simulink model "actuador_modelo_global_NL"  (R2023b)
settings: Solver=VariableStepAuto  StartTime=0.0  StopTime=10.0  RelTol=1e-3
values from neighbouring files (symbols this model uses):
  alpha_Cu = 3.9e-3    (= 0.0039)    [controlador_foc_simulink.m]    (also in parametros_planta.m; params_subsistema_termico.m; sistema_completo_en_codigo.m)
  beq_nom = bm + bl_nom/r^2    (= 2.19444444444e-05)    [parametros_planta.m]    (also in params_subsistema_mecanico.m; sistema_completo_en_codigo.m)
  Cts = 0.818    [parametros_planta.m]    (also in params_subsistema_termico.m)
  Jeq_nom = Jm + Jl_nom/r^2    (= 1.97847222222e-05)    [params_subsistema_mecanico.m]    (also in sistema_completo_en_codigo.m)
  kg_eq_nom = g*kl_nom/r    (= 0.0204305208333)    [params_subsistema_mecanico.m]    (also in sistema_completo_en_codigo.m)
  L_d = 6.6e-3    (= 0.0066)    [controlador_foc_simulink.m]    (also in params_subsistema_electromagnetico.m; sistema_completo_en_codigo.m)
  L_l = 0.8e-3    (= 0.0008)    [controlador_foc_simulink.m]    (also in params_subsistema_electromagnetico.m; sistema_completo_en_codigo.m)
  L_q = 5.8e-3    (= 0.0058)    [controlador_foc_simulink.m]    (also in params_subsistema_electromagnetico.m; sistema_completo_en_codigo.m)
  lambda_m = 0.016    [controlador_foc_simulink.m]    (also in parametros_planta.m; params_subsistema_electromagnetico.m; sistema_completo_en_codigo.m)
  Pp = 3    [controlador_foc_simulink.m]    (also in parametros_planta.m; params_subsistema_electromagnetico.m; sistema_completo_en_codigo.m)
  r = 120.0    (= 120)    [controlador_foc_simulink.m]    (also in parametros_planta.m; params_subsistema_mecanico.m; sistema_completo_en_codigo.m)
  Rs_REF = 1.02    [controlador_foc_simulink.m]    (also in parametros_planta.m; params_subsistema_termico.m; sistema_completo_en_codigo.m)
  Rts_amb = 146.7    [parametros_planta.m]    (also in params_subsistema_termico.m)
  Tamb = Tamb_max    (= 40)    [parametros_planta.m]    (also in params_subsistema_termico.m; sistema_completo_en_codigo.m)
  Ts_REF = 20.0    (= 20)    [controlador_foc_simulink.m]    (also in parametros_planta.m; params_subsistema_termico.m; sistema_completo_en_codigo.m)
settings Model: Creator=Pc  LastModifiedBy=Gabriel

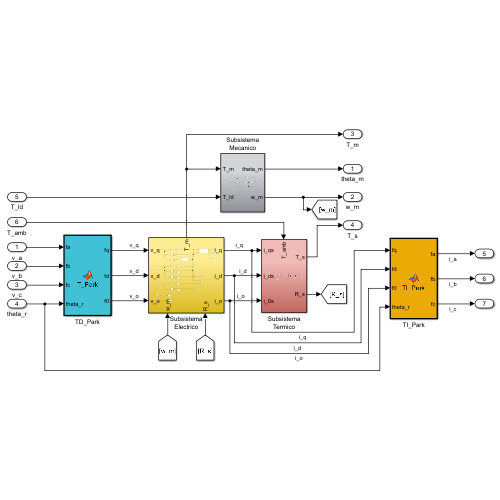
[thumbnail: Simulink's stored preview of the top-level diagram]
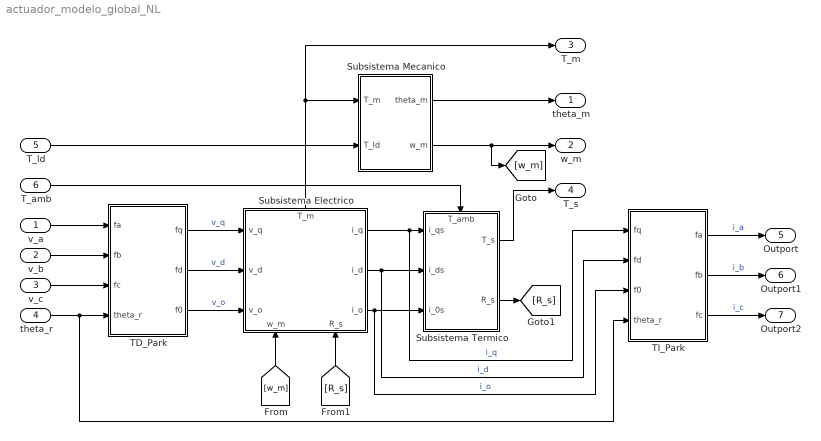
== system actuador_modelo_global_NL ==
  v_a : Inport
  v_b : Inport  Port=2
  v_c : Inport  Port=3
  theta_r : Inport  Port=4
  T_ld : Inport  Port=5
  T_amb : Inport  Port=6
  Subsistema Electrico : Subsystem
      settings: PortSchema="{\"entries\":[{\"content\":{\"sides\":[{\"content\":{\"connectorIds\":[\"In1\",\"In2\",\"In3\"]},\"type\":\"ConnectorPlacement.EquallySpacedRectSide\",\"uuid\":\"c7eb63ae-4015-4be9-a2f8-5ddbad38e871\"},{\"content\":{\"connectorIds\":[\"Out1\",\"Out2\",\"Out3\"],\"side\":\"RIGHT\"},\"type\":\"ConnectorPlacement.EquallySpacedRectSide\",\"uuid\":\"ed205027-9864-417a-9d2b-6eeb723ffec2\"},{\"content\":{\"connectorIds\":[\"Out4\"],\"side\":\"TOP\"},\"type\":\"ConnectorPlacement.EquallySpacedRectSide\",\"uuid\":\"5c5dee03-5728-4212-8fc2-a453d3484329\"},{\"content\":{\"connectorIds\":[\"In4\",\"In5\"],\"side\":\"BOTTOM\"},\"type\":\"ConnectorPlacement.EquallySpacedRectSide\",\"uuid\":\"494df340-b6d5-4f09-932e-9dbff39af1cf\"}]},\"type\":\"ConnectorPlacement.EquallySpacedConnector\",\"uuid\":\"0eeaea4c-3d80-4ebb-8c27-59b1b18764e9\"}],\"packageUris\":[\"http://schema.mathworks.com/mf0/Connector/R2020b\"],\"version\":\"1.0\"}"
  Subsistema Mecanico : Subsystem
  Subsistema Termico : Subsystem
      settings: PortSchema="{\"entries\":[{\"content\":{\"sides\":[{\"content\":{\"connectorIds\":[\"In1\",\"In2\",\"In3\"]},\"type\":\"ConnectorPlacement.EquallySpacedRectSide\",\"uuid\":\"5b1848a7-84bd-4673-a3fa-3976b4d0d5b9\"},{\"content\":{\"connectorIds\":[\"Out1\",\"Out2\"],\"side\":\"RIGHT\"},\"type\":\"ConnectorPlacement.EquallySpacedRectSide\",\"uuid\":\"feff3f8a-cd7c-43b1-91c3-7ab01b0b33a6\"},{\"content\":{\"connectorIds\":[\"In4\"],\"side\":\"TOP\"},\"type\":\"ConnectorPlacement.EquallySpacedRectSide\",\"uuid\":\"8de0b1b6-142f-442a-a92f-2baa615c6322\"}]},\"type\":\"ConnectorPlacement.EquallySpacedConnector\",\"uuid\":\"046fcb24-e0d9-4784-a784-7e36f9acbfbc\"}],\"packageUris\":[\"http://schema.mathworks.com/mf0/Connector/R2020b\"],\"version\":\"1.0\"}"
  TD_Park : MATLAB Function  TreatAsAtomicUnit=on
  TI_Park : MATLAB Function  TreatAsAtomicUnit=on
  theta_m : Outport
  w_m : Outport  Port=2
  T_m : Outport  Port=3
  T_s : Outport  Port=4
  Outport : Outport  Port=5
  Outport1 : Outport  Port=6
  Outport2 : Outport  Port=7
  wires:
  Subsistema Electrico/1(i_q) -> TI_Park/1(fq), Subsistema Termico/1(i_qs)  "i_q"
  Subsistema Electrico/2(i_d) -> Subsistema Termico/2(i_ds), TI_Park/2(fd)  "i_d"
  Subsistema Electrico/3(i_o) -> Subsistema Termico/3(i_0s), TI_Park/3(f0)  "i_o"
  TD_Park/1(fq) -> Subsistema Electrico/1(v_q)  "v_q"
  TD_Park/2(fd) -> Subsistema Electrico/2(v_d)  "v_d"
  TD_Park/3(f0) -> Subsistema Electrico/3(v_o)  "v_o"
  T_amb/1 -> Subsistema Termico/4(T_amb)
  Subsistema Mecanico/2(w_m) -> [w_m], w_m/1
  Subsistema Mecanico/1(theta_m) -> theta_m/1
  v_a/1 -> TD_Park/1(fa)
  v_b/1 -> TD_Park/2(fb)
  v_c/1 -> TD_Park/3(fc)
  Subsistema Termico/1(T_s) -> T_s/1
  theta_r/1 -> TI_Park/4(theta_r), TD_Park/4(theta_r)
  Subsistema Electrico/4(T_m) -> T_m/1, Subsistema Mecanico/1(T_m)
  T_ld/1 -> Subsistema Mecanico/2(T_ld)
  [w_m] -> Subsistema Electrico/4(w_m)
  Subsistema Termico/2(R_s) -> [R_s]
  [R_s] -> Subsistema Electrico/5(R_s)
  TI_Park/1(fa) -> Outport/1  "i_a"
  TI_Park/2(fb) -> Outport1/1  "i_b"
  TI_Park/3(fc) -> Outport2/1  "i_c"

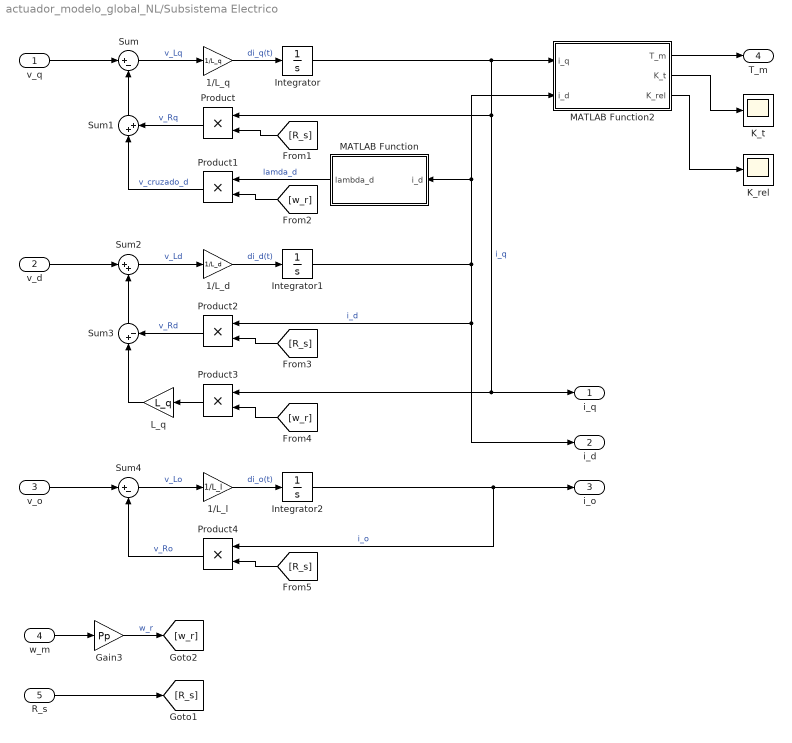
== system actuador_modelo_global_NL/Subsistema Electrico ==
  v_q : Inport
  v_d : Inport  Port=2
  v_o : Inport  Port=3
  w_m : Inport  Port=4
  R_s : Inport  Port=5
  1/L_d : Gain  Gain=1/L_d
  1/L_l : Gain  Gain=1/L_l
  1/L_q : Gain  Gain=1/L_q
  Gain3 : Gain  Gain=Pp
  Integrator : Integrator
  Integrator1 : Integrator
  Integrator2 : Integrator
  K_rel : Scope
  K_t : Scope
  L_q : Gain  Gain=L_q
  MATLAB Function : MATLAB Function  TreatAsAtomicUnit=on
  MATLAB Function2 : MATLAB Function  TreatAsAtomicUnit=on
  Product{,1..4} (5 alike) : Product
  Sum : Sum  Inputs=|+-
  Sum1 : Sum  Inputs=|++
  Sum2 : Sum  Inputs=|++
  Sum3 : Sum  Inputs=|+-
  Sum4 : Sum  Inputs=|+-
  i_q : Outport
  i_d : Outport  Port=2
  i_o : Outport  Port=3
  T_m : Outport  Port=4
  wires:
  Integrator/1 -> MATLAB Function2/1(i_q), Product/1, i_q/1, Product3/1  "i_q"
  Sum3/1 -> Sum2/2
  Product1/1 -> Sum1/1  "v_cruzado_d"
  Integrator1/1 -> MATLAB Function2/2(i_d), MATLAB Function/1(i_d), i_d/1, Product2/1  "i_d"
  Sum1/1 -> Sum/2
  1/L_d/1 -> Integrator1/1  "di_d(t)"
  MATLAB Function/1(lambda_d) -> Product1/1  "lamda_d"
  Sum4/1 -> 1/L_l/1  "v_Lo"
  [w_r] -> Product3/2
  Sum/1 -> 1/L_q/1  "v_Lq"
  1/L_l/1 -> Integrator2/1  "di_o(t)"
  Integrator2/1 -> i_o/1, Product4/1  "i_o"
  Product2/1 -> Sum3/2  "v_Rd"
  Product/1 -> Sum1/2  "v_Rq"
  [R_s] -> Product4/2
  Product3/1 -> L_q/1
  1/L_q/1 -> Integrator/1  "di_q(t)"
  Sum2/1 -> 1/L_d/1  "v_Ld"
  v_q/1 -> Sum/1
  [R_s] -> Product/2
  Product4/1 -> Sum4/2  "v_Ro"
  [w_r] -> Product1/2
  [R_s] -> Product2/2
  L_q/1 -> Sum3/1
  v_d/1 -> Sum2/1
  v_o/1 -> Sum4/1
  MATLAB Function2/1(T_m) -> T_m/1
  MATLAB Function2/3(K_rel) -> K_rel/1
  MATLAB Function2/2(K_t) -> K_t/1
  w_m/1 -> Gain3/1
  R_s/1 -> [R_s]
  Gain3/1 -> [w_r]  "w_r"

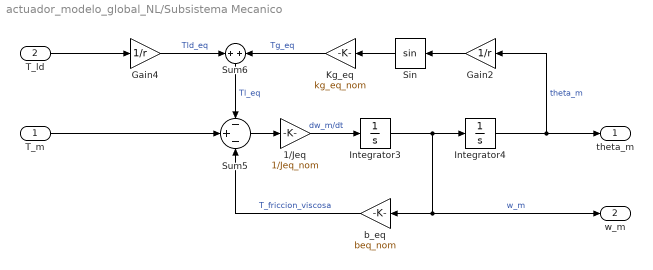
== system actuador_modelo_global_NL/Subsistema Mecanico ==
  T_m : Inport
  T_ld : Inport  Port=2
  1/Jeq : Gain  Gain=1/Jeq_nom
  Gain2 : Gain  Gain=1/r
  Gain4 : Gain  Gain=1/r
  Integrator3 : Integrator
  Integrator4 : Integrator
  Kg_eq : Gain  Gain=kg_eq_nom
  Sin : Trigonometry
  Sum5 : Sum  Inputs=-+-
  Sum6 : Sum  Inputs=+|+
  b_eq : Gain  Gain=beq_nom
  theta_m : Outport
  w_m : Outport  Port=2
  wires:
  Sin/1 -> Kg_eq/1
  Gain4/1 -> Sum6/1  "Tld_eq"
  Integrator4/1 -> theta_m/1, Gain2/1  "theta_m"
  Kg_eq/1 -> Sum6/2  "Tg_eq"
  Sum5/1 -> 1/Jeq/1
  b_eq/1 -> Sum5/3  "T_friccion_viscosa"
  T_m/1 -> Sum5/2
  Gain2/1 -> Sin/1
  Sum6/1 -> Sum5/1  "Tl_eq"
  Integrator3/1 -> w_m/1, b_eq/1, Integrator4/1  "w_m"
  T_ld/1 -> Gain4/1
  1/Jeq/1 -> Integrator3/1  "dw_m/dt"

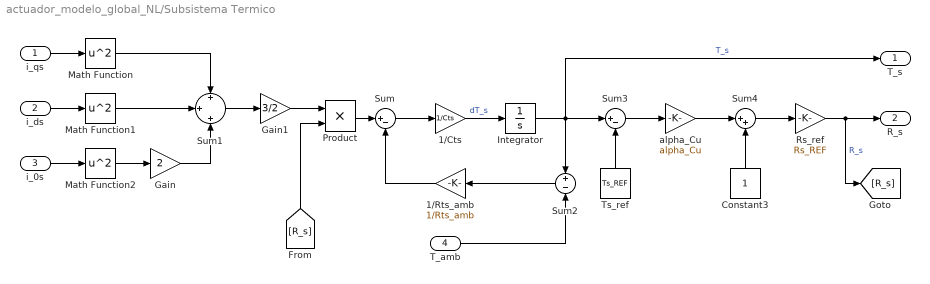
== system actuador_modelo_global_NL/Subsistema Termico ==
  i_qs : Inport
  i_ds : Inport  Port=2
  i_0s : Inport  Port=3
  T_amb : Inport  Port=4
  1/Cts : Gain  Gain=1/Cts
  1/Rts_amb : Gain  Gain=1/Rts_amb
  Constant3 : Constant
  Gain : Gain  Gain=2
  Gain1 : Gain  Gain=3/2
  Integrator : Integrator  InitialCondition=Tamb
  Math Function : Math  Operator=square
  Math Function1 : Math  Operator=square
  Math Function2 : Math  Operator=square
  Product : Product
  Rs_ref : Gain  Gain=Rs_REF
  Sum : Sum  Inputs=|+-
  Sum1 : Sum  Inputs=+|+|+
  Sum2 : Sum  Inputs=+-
  Sum3 : Sum  Inputs=|+-
  Sum4 : Sum  Inputs=|++
  Ts_ref : Constant  Value=Ts_REF
  alpha_Cu : Gain  Gain=alpha_Cu
  T_s : Outport
  R_s : Outport  Port=2
  wires:
  1/Cts/1 -> Integrator/1  "dT_s"
  Sum3/1 -> alpha_Cu/1
  Rs_ref/1 -> R_s/1, [R_s]  "R_s"
  Sum4/1 -> Rs_ref/1
  [R_s] -> Product/2
  i_ds/1 -> Math Function1/1
  Constant3/1 -> Sum4/2
  Integrator/1 -> T_s/1, Sum2/1, Sum3/1  "T_s"
  Math Function1/1 -> Sum1/2
  alpha_Cu/1 -> Sum4/1
  Sum2/1 -> 1/Rts_amb/1
  Product/1 -> Sum/1
  i_qs/1 -> Math Function/1
  Sum/1 -> 1/Cts/1
  T_amb/1 -> Sum2/2
  Math Function/1 -> Sum1/1
  i_0s/1 -> Math Function2/1
  1/Rts_amb/1 -> Sum/2
  Ts_ref/1 -> Sum3/2
  Math Function2/1 -> Gain/1
  Gain/1 -> Sum1/3
  Sum1/1 -> Gain1/1
  Gain1/1 -> Product/1

== matlab function actuador_modelo_global_NL/TD_Park ==
  data: fa input; fq output; fb input; fc input; theta_r input; fd output; f0 output
function [fq, fd, f0] = T_Park(fa, fb, fc, theta_r)
%#codegen
% Transformada directa de Park: abc -> qd0
% Convención usada:
% fq: eje q
% fd: eje d
% f0: componente homopolar

c1 = cos(theta_r);
c2 = cos(theta_r - 2*pi/3);
c3 = cos(theta_r + 2*pi/3);

s1 = sin(theta_r);
s2 = sin(theta_r - 2*pi/3);
s3 = sin(theta_r + 2*pi/3);

fq = (2/3)*(c1*fa + c2*fb + c3*fc);
fd = (2/3)*(s1*fa + s2*fb + s3*fc);
f0 = (1/3)*(fa + fb + fc);
end

== matlab function actuador_modelo_global_NL/Subsistema Electrico/MATLAB Function ==
  data: i_d input; lambda_d output; lambda_m parameter; L_d parameter
function lambda_d = calcular_flujo_d(i_d, lambda_m, L_d)
    % CALCULAR_FLUJO_D Calcula el flujo magnético total concatenado en el eje directo (d).
    %
    % Entradas:
    %   i_d      : Corriente instantánea en el eje d (Señal dinámica de entrada).
    %   lambda_m : Flujo de los imanes permanentes (Parámetro estático).
    %   L_d      : Inductancia del estator en el eje d (Parámetro estático).
    %
    % Salida:
    %   lambda_d : Flujo magnético total en el eje d.

    % Cálculo: Flujo de imanes + Flujo de reacción del inducido
    lambda_d = lambda_m + L_d * i_d;
end

== matlab function actuador_modelo_global_NL/Subsistema Electrico/MATLAB Function2 ==
  data: i_q input; i_d input; T_m output; Pp parameter; lambda_m parameter; L_d parameter; L_q parameter; K_t output; K_rel output
function [T_m, K_t, K_rel] = calcular_torque(i_q, i_d, Pp, lambda_m, L_d, L_q)
    % CALCULAR_TORQUE Calcula el torque electromagnético total de la máquina PMSM
    % y sus constantes equivalentes.
    % 
    % Entradas dinámicas (Inports):
    %   i_q      : Corriente en el eje en cuadratura [A].
    %   i_d      : Corriente en el eje directo [A].
    %
    % Parámetros estáticos (Parameters):
    %   P_p      : Número de pares de polos.
    %   lambda_m : Flujo magnético de los imanes permanentes [Wb].
    %   L_d      : Inductancia del eje d [H].
    %   L_q      : Inductancia del eje q [H].
    %
    % Salidas:
    %   T_m      : Torque electromagnético generado [N.m].
    %   K_t      : Constante de torque de alineación [N.m/A].
    %   K_rel    : Constante de torque de reluctancia [N.m/A^2].

    % 1. Cálculo de las constantes 
    K_t = (3/2) * Pp * lambda_m;
    K_rel = (3/2) * Pp * (L_d - L_q);

    % 2. Cálculo del torque electromagnético total
    T_m = K_t * i_q + K_rel * i_d * i_q;
end

== matlab function actuador_modelo_global_NL/TI_Park ==
  data: fq input; fa output; fd input; f0 input; theta_r input; fb output; fc output
function [fa, fb, fc] = TI_Park(fq, fd, f0, theta_r)
%#codegen
% Transformada inversa de Park: qd0 -> abc

fa = cos(theta_r)*fq ...
   + sin(theta_r)*fd ...
   + f0;

fb = cos(theta_r - 2*pi/3)*fq ...
   + sin(theta_r - 2*pi/3)*fd ...
   + f0;

fc = cos(theta_r + 2*pi/3)*fq ...
   + sin(theta_r + 2*pi/3)*fd ...
   + f0;
end
